simulink model "Uklad_wersja_Liniowa_Schemat"  (R2018a)
settings: Solver=VariableStepAuto  StartTime=0.0  StopTime=10.0  RelTol=1e-3
values from neighbouring files (symbols this model uses):
  A1 = 1    [Uklad_Wersja_Laczna.m]    (also in Uklad_wersja_Liniowa.m; Uklad_wersja_Nieliniowa.m; test.m)
  a1 = Aw1*sqrt(2*g)    [Uklad_Wersja_Laczna.m]    (also in Uklad_wersja_Liniowa.m = 1)
  A2 = 1    [Uklad_Wersja_Laczna.m]    (also in Uklad_wersja_Liniowa.m; Uklad_wersja_Nieliniowa.m; test.m)
  a2 = Aw2*sqrt(2*g)    [Uklad_Wersja_Laczna.m]    (also in Uklad_wersja_Liniowa.m = 1)
  dfew1 = 0.1*fwe_max    [Uklad_Wersja_Laczna.m]    (also in Uklad_wersja_Liniowa.m = 0; Uklad_wersja_Nieliniowa.m = 1; test.m = 1)
  fwe1 = f(i)    [Uklad_Wersja_Laczna.m]    (also in Uklad_wersja_Liniowa.m = 1; Uklad_wersja_Nieliniowa.m = 1; test.m = 0)
  h10 = 1    [Uklad_Wersja_Laczna.m]    (also in Uklad_wersja_Liniowa.m = 3; Uklad_wersja_Nieliniowa.m = 5.09683995923; test.m = 0.6)
  h20 = 1    [Uklad_Wersja_Laczna.m]    (also in Uklad_wersja_Liniowa.m = 2; Uklad_wersja_Nieliniowa.m = 1.27420998981; test.m = 2)
settings Model: Creator=john  LastModifiedBy=john

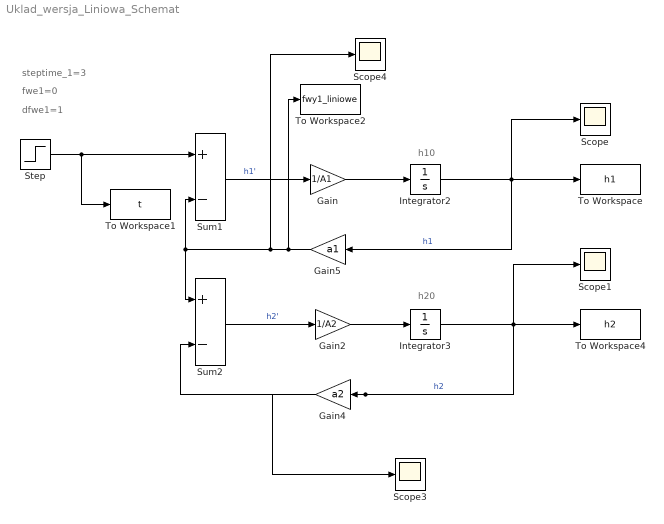
== system Uklad_wersja_Liniowa_Schemat ==
  note: dfwe1=1
  note: fwe1=0
  note: h10
  note: steptime_1=3
  note: h20
  Gain : Gain  Gain=1/A1
  Gain2 : Gain  Gain=1/A2
  Gain4 : Gain  Gain=a2
  Gain5 : Gain  Gain=a1
  Integrator2 : Integrator  InitialCondition=h10
  Integrator3 : Integrator  InitialCondition=h20
  Scope{,1,3..4} (4 alike) : Scope
  Step : Step  Time=0  Before=fwe1  After=dfew1+fwe1  SampleTime=0
  Sum1 : Sum  Inputs=+-
  Sum2 : Sum  Inputs=+-
  To Workspace : ToWorkspace  VariableName=h1  SampleTime=-1
  To Workspace1 : ToWorkspace  VariableName=t  SaveFormat=Timeseries  SampleTime=-1
  To Workspace2 : ToWorkspace  VariableName=fwy1_liniowe  SampleTime=-1
  To Workspace4 : ToWorkspace  VariableName=h2  SampleTime=-1
  wires:
  Integrator3/1 -> Scope3/1, Gain4/1, Scope1/1, To Workspace4/1  "h2"
  Gain/1 -> Integrator2/1
  Integrator2/1 -> Gain5/1, To Workspace/1, Scope/1  "h1"
  Gain4/1 -> Sum2/2
  Gain2/1 -> Integrator3/1
  Sum2/1 -> Gain2/1  "h2'"
  Step/1 -> To Workspace1/1, Sum1/1
  Sum1/1 -> Gain/1  "h1'"
  Gain5/1 -> To Workspace2/1, Scope4/1, Sum2/1, Sum1/2
